simulink subsystem "Lazo_Corrientes"  (R2026a)
settings: Solver=VariableStepAuto
values from neighbouring files (symbols this model uses):
  Pp = 3    [coeficientes.m]
  R0 = abs(p)*L_ls    [coeficientes.m]
  Rd = abs(p)*L_d    [coeficientes.m]
  Rq = abs(p)*L_q    [coeficientes.m]
libraries: eeTransforms x1
settings Model: Creator=admin  LastModifiedBy=admin

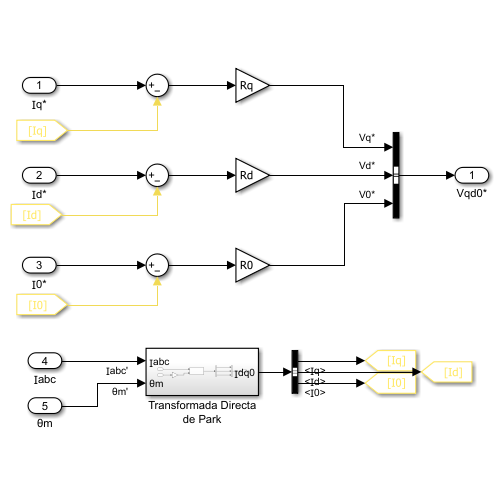
[thumbnail: Simulink's stored preview of the top-level diagram]
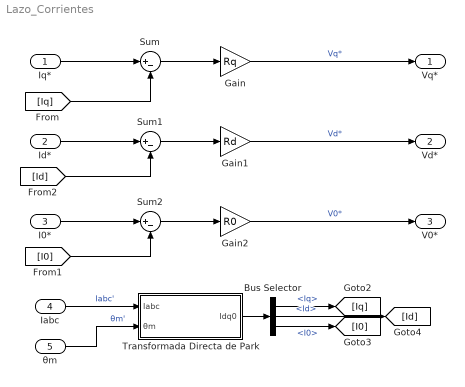
== system Lazo_Corrientes ==
  Ⅰq* : Inport
  Ⅰd* : Inport  Port=2
  Ⅰ0* : Inport  Port=3
  Ⅰabc : Inport  Port=4
  θm : Inport  Port=5
  Bus Selector : BusSelector  OutputSignals=Ⅰq,Ⅰd,Ⅰ0
  Gain : Gain  Gain=Rq
  Gain1 : Gain  Gain=Rd
  Gain2 : Gain  Gain=R0
  Sum : Sum  Inputs=|+-
  Sum1 : Sum  Inputs=|+-
  Sum2 : Sum  Inputs=|+-
  Transformada Directa de Park : Subsystem
  Vq* : Outport
  Vd* : Outport  Port=2
  V0* : Outport  Port=3
  wires:
  Bus Selector/1 -> [Iq]  "<Ⅰq>"
  θm/1 -> Transformada Directa de Park/2(θm)  "θm'"
  Ⅰabc/1 -> Transformada Directa de Park/1(Ⅰabc)  "Ⅰabc'"
  Transformada Directa de Park/1(Ⅰdq0) -> Bus Selector/1
  Bus Selector/3 -> [I0]  "<Ⅰ0>"
  Bus Selector/2 -> [Id]  "<Ⅰd>"
  Ⅰq*/1 -> Sum/1
  [Iq] -> Sum/2
  Ⅰd*/1 -> Sum1/1
  [Id] -> Sum1/2
  Ⅰ0*/1 -> Sum2/1
  [I0] -> Sum2/2
  Sum2/1 -> Gain2/1
  Sum1/1 -> Gain1/1
  Sum/1 -> Gain/1
  Gain/1 -> Vq*/1  "Vq*"
  Gain1/1 -> Vd*/1  "Vd*"
  Gain2/1 -> V0*/1  "V0*"

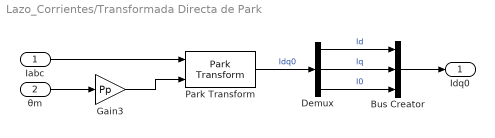
== system Lazo_Corrientes/Transformada Directa de Park ==
  Ⅰabc : Inport
  θm : Inport  Port=2
  Bus Creator : BusCreator  Inputs=3
  Demux : Demux  Outputs=3
  Gain3 : Gain  Gain=Pp
  Park Transform : eeTransforms/Park Transform  AxisAlignment=Q-axis  PowerInvariant=off
      settings: LibrarySourceBlock=|
      | ee_sl_lib/Mathematical
      | Transforms/Park Transform
  Ⅰdq0 : Outport
  wires:
  Gain3/1 -> Park Transform/2
  Park Transform/1 -> Demux/1  "Ⅰdq0"
  Demux/1 -> Bus Creator/1  "Ⅰd"
  Demux/3 -> Bus Creator/3  "Ⅰ0"
  Demux/2 -> Bus Creator/2  "Ⅰq"
  Bus Creator/1 -> Ⅰdq0/1
  Ⅰabc/1 -> Park Transform/1
  θm/1 -> Gain3/1
